simulink model "CounterUpDown_RE_test"  (R2013a)
settings: Solver=ode3  StartTime=0.0  StopTime=10  RelTol=1e-3
libraries: simulink_extras x2, PTC_MBDS_LIB x1
settings Model: Creator=kyle.willis  LastModifiedBy=kyle.willis
settings OptimizationCC: InlineParams=on

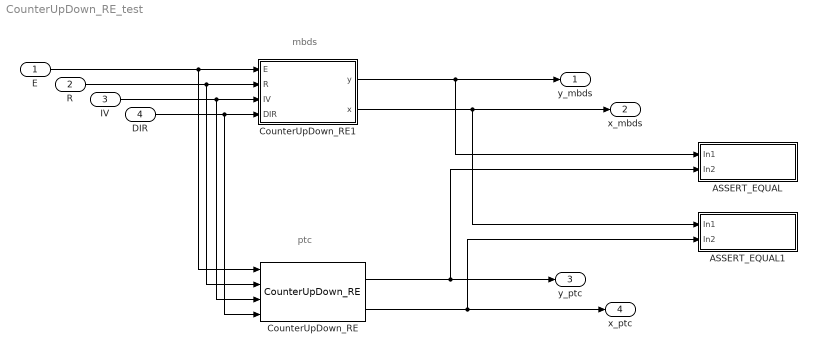
== system CounterUpDown_RE_test ==
  note: ptc
  note: mbds
  E : Inport
  R : Inport  Port=2
  IV : Inport  Port=3
  DIR : Inport  Port=4
  ASSERT_EQUAL : Subsystem
  ASSERT_EQUAL1 : Subsystem
  CounterUpDown_RE : PTC_MBDS_LIB/MBDS Standard Library/Extended Operations/Counter & Timer/CounterUpDown_RE  E_Enabled=on  R_Enabled=on  IV_Enabled=on  IV=0  y_Enabled=on  x_Enabled=on  OutDataTypeStr=Inherit: Inherit via back propagation  PTC_MBDS_BlockVersion=5.40  PTC_BlockType=PTC_MBDS_CounterUpDown_RE
  CounterUpDown_RE1 : Subsystem  InitFcn=|  mask(CounterUpDown_RE){MBDS_LibraryBlock=on, E_Enabled=on, R_Enabled=on, IV_Enabled=on, IV=0, y_Enabled=on, x_Enabled=on, OutDataTypeStr=Inherit: Inherit via back propagation, MBDS_BlockVersion=05.40}
      | if(exist('MBDS_BlockCallback', 'file'))
      |    MBDS_BlockCallback('Update', gcb);
      | end
      mask prompts: MBDS_LibraryBlock "MBDS library block"; E_Enabled "Show E port"; R_Enabled "Show R port"; IV_Enabled "Show IV port"; IV "Initial value (IV):"; y_Enabled "Show y port"; x_Enabled "Show x port"; OutDataTypeStr "Output data type:"; MBDS_BlockVersion "Block version:"
      mask help: This block provides a counter where the direction of counting (up or down) can be controlled by an input port.
      mask init:
      | if(exist('MBDS_BlockCallback', 'file'))
      |    MBDS_BlockCallback('Init', gcb);
      | else
      |    % Disable all mask parameters
      |    MaskEnables = get_param(gcb, 'MaskEnables');
      |    for k = [1:length(MaskEnables)]
      |       MaskEnables{k} = 'off';
      |    end
      |    if(~isequal(MaskEnables, get_param(gcb, 'MaskEnables')))
      |       set_param(gcb, 'MaskEnables', MaskEnables);
      |    end
      | end
      mask Help: eval(['open([workdir(''library_dir:''),''\Blockset\help\'',get_param(gcb,''MaskType''),''.html''])'])
      mask Callback R_Enabled:
      | % Update mask parameter dialog
      | if(exist('MBDS_BlockCallback', 'file'))
      |    MBDS_BlockCallback('R_Enabled', gcb);
      | end
      mask Callback IV_Enabled:
      | % Update mask parameter dialog
      | if(exist('MBDS_BlockCallback', 'file'))
      |    MBDS_BlockCallback('IV_Enabled', gcb);
      | end
      mask Callback IV:
      | % Adopt Value
      | if(exist('MBDS_BlockCallback', 'file'))
      |    MBDS_BlockCallback('IV', gcb);
      | end
      mask Callback y_Enabled:
      | % Update mask parameter dialog
      | if(exist('MBDS_BlockCallback', 'file'))
      |    MBDS_BlockCallback('y_Enabled', gcb);
      | end
      mask Callback x_Enabled:
      | % Update mask parameter dialog
      | if(exist('MBDS_BlockCallback', 'file'))
      |    MBDS_BlockCallback('x_Enabled', gcb);
      | end
      mask TypeOptions OutDataTypeStr: Inherit: Inherit via back propagation | int8 | uint8 | int16 | uint16 | int32 | uint32
      mask Callback OutDataTypeStr:
      | % Configure data type
      | if(exist('MBDS_BlockCallback', 'file'))
      |    MBDS_BlockCallback('OutDataTypeStr', gcb);
      | end
      mask Display:
      | % Show icon or block text
      | if(exist('CounterUpDown.tif', 'file'))
      |    image(imread('CounterUpDown.tif','tif'), [0.295739348370927 0.225 0.378947368421053 0.55]);
      |    disp('')
      | else
      |    disp(sprintf('Count\nUp/Down'));
      | end
      | 
      | % Display port labels
      | port_label('input', 1, 'E');
      | port_label('input', 2, 'R');
      | port_label('input', 3, 'IV');
      | port_label('input', 4, 'DIR');
      | port_label('output', 1, 'y');
      | port_label('output', 2, 'x');
  y_mbds : Outport
  x_mbds : Outport  Port=2
  y_ptc : Outport  Port=3
  x_ptc : Outport  Port=4
  wires:
  E/1 -> CounterUpDown_RE1/1(E), CounterUpDown_RE/1
  R/1 -> CounterUpDown_RE1/2(R), CounterUpDown_RE/2
  IV/1 -> CounterUpDown_RE1/3(IV), CounterUpDown_RE/3
  CounterUpDown_RE1/1(y) -> ASSERT_EQUAL/1(In1), y_mbds/1
  CounterUpDown_RE1/2(x) -> x_mbds/1, ASSERT_EQUAL1/1(In1)
  CounterUpDown_RE/1 -> ASSERT_EQUAL/2(In2), y_ptc/1
  CounterUpDown_RE/2 -> ASSERT_EQUAL1/2(In2), x_ptc/1
  DIR/1 -> CounterUpDown_RE1/4(DIR), CounterUpDown_RE/4

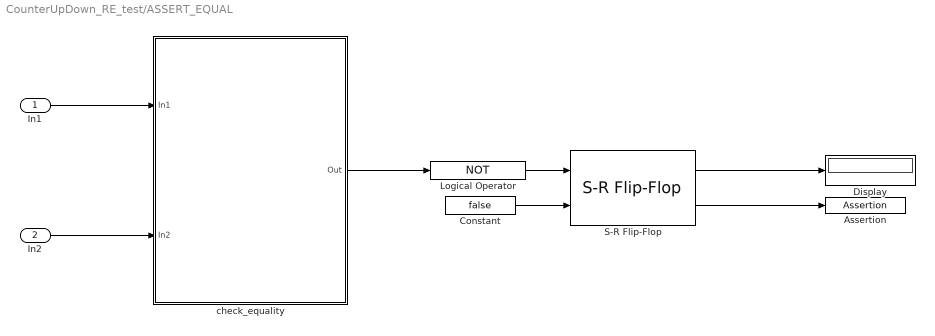
== system CounterUpDown_RE_test/ASSERT_EQUAL ==
  In1 : Inport
  In2 : Inport  Port=2
  Assertion : Assertion
  Constant : Constant  Value=false
  Display : Display
  Logical Operator : Logic  Operator=NOT  AllPortsSameDT=off  OutDataTypeStr=boolean
  S-R Flip-Flop : simulink_extras/Flip Flops/S-R Flip-Flop  initial_condition=0
  check_equality : MATLAB Function  TreatAsAtomicUnit=on
  wires:
  S-R Flip-Flop/1 -> Display/1
  check_equality/1(Out) -> Logical Operator/1
  Constant/1 -> S-R Flip-Flop/2
  S-R Flip-Flop/2 -> Assertion/1
  In2/1 -> check_equality/2(In2)
  In1/1 -> check_equality/1(In1)
  Logical Operator/1 -> S-R Flip-Flop/1

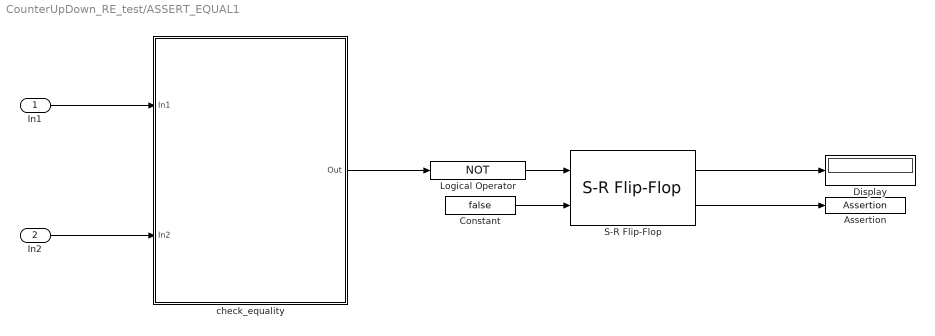
== system CounterUpDown_RE_test/ASSERT_EQUAL1 ==
  In1 : Inport
  In2 : Inport  Port=2
  Assertion : Assertion
  Constant : Constant  Value=false
  Display : Display
  Logical Operator : Logic  Operator=NOT  AllPortsSameDT=off  OutDataTypeStr=boolean
  S-R Flip-Flop : simulink_extras/Flip Flops/S-R Flip-Flop  initial_condition=0
  check_equality : MATLAB Function  TreatAsAtomicUnit=on
  wires:
  Logical Operator/1 -> S-R Flip-Flop/1
  In1/1 -> check_equality/1(In1)
  In2/1 -> check_equality/2(In2)
  S-R Flip-Flop/2 -> Assertion/1
  Constant/1 -> S-R Flip-Flop/2
  check_equality/1(Out) -> Logical Operator/1
  S-R Flip-Flop/1 -> Display/1

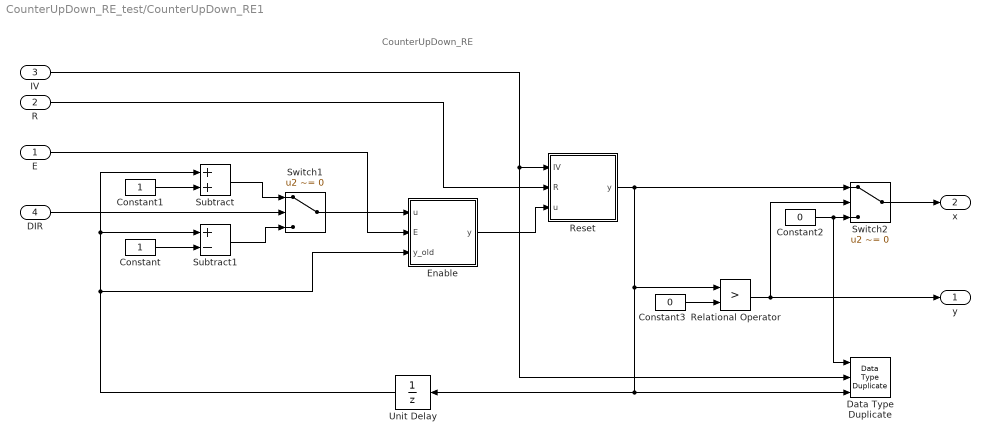
== system CounterUpDown_RE_test/CounterUpDown_RE1 ==
  note: CounterUpDown_RE
  E : Inport  OutDataTypeStr=boolean
  R : Inport  Port=2  OutDataTypeStr=boolean
  IV : Inport  Port=3
  DIR : Inport  Port=4  OutDataTypeStr=boolean
  Constant : Constant  OutDataTypeStr=Inherit: Inherit via back propagation
  Constant1 : Constant  OutDataTypeStr=Inherit: Inherit via back propagation
  Constant2 : Constant  Value=0  OutDataTypeStr=Inherit: Inherit via back propagation
  Constant3 : Constant  Value=0  OutDataTypeStr=Inherit: Inherit via back propagation
  Data Type Duplicate : DataTypeDuplicate  NumInputPorts=3
  Enable : Subsystem
  Relational Operator : RelationalOperator  Operator=>  OutDataTypeStr=boolean  InputSameDT=on
  Reset : Subsystem
  Subtract : Sum  OutDataTypeStr=Inherit: Inherit via back propagation  SaturateOnIntegerOverflow=on  InputSameDT=on
  Subtract1 : Sum  Inputs=+-  OutDataTypeStr=Inherit: Inherit via back propagation  SaturateOnIntegerOverflow=on  InputSameDT=on
  Switch1 : Switch  Criteria=u2 ~= 0  OutDataTypeStr=Inherit: Inherit via back propagation  InputSameDT=on
  Switch2 : Switch  Criteria=u2 ~= 0  OutDataTypeStr=Inherit: Inherit via back propagation  InputSameDT=on
  Unit Delay : UnitDelay  SampleTime=-1
  y : Outport
  x : Outport  Port=2
  wires:
  DIR/1 -> Switch1/2
  R/1 -> Reset/2(R)
  E/1 -> Enable/2(E)
  Subtract/1 -> Switch1/1
  Subtract1/1 -> Switch1/3
  Constant/1 -> Subtract1/2
  Constant1/1 -> Subtract/2
  Switch1/1 -> Enable/1(u)
  Relational Operator/1 -> Switch2/2, y/1
  IV/1 -> Data Type Duplicate/2, Reset/1(IV)
  Switch2/1 -> x/1
  Constant3/1 -> Relational Operator/2
  Constant2/1 -> Switch2/3, Data Type Duplicate/1
  Unit Delay/1 -> Enable/3(y_old), Subtract1/1, Subtract/1
  Reset/1(y) -> Unit Delay/1, Data Type Duplicate/3, Relational Operator/1, Switch2/1
  Enable/1(y) -> Reset/3(u)

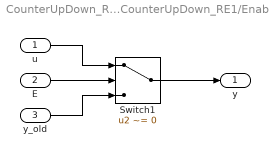
== system CounterUpDown_RE_test/CounterUpDown_RE1/Enable ==
  u : Inport
  E : Inport  Port=2
  y_old : Inport  Port=3
  Switch1 : Switch  Criteria=u2 ~= 0  OutDataTypeStr=Inherit: Inherit via back propagation  InputSameDT=on
  y : Outport
  wires:
  y_old/1 -> Switch1/3
  Switch1/1 -> y/1
  u/1 -> Switch1/1
  E/1 -> Switch1/2

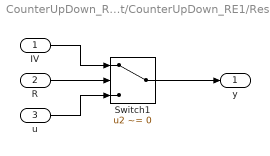
== system CounterUpDown_RE_test/CounterUpDown_RE1/Reset ==
  IV : Inport
  R : Inport  Port=2
  u : Inport  Port=3
  Switch1 : Switch  Criteria=u2 ~= 0  OutDataTypeStr=Inherit: Inherit via back propagation  InputSameDT=on
  y : Outport
  wires:
  u/1 -> Switch1/3
  Switch1/1 -> y/1
  IV/1 -> Switch1/1
  R/1 -> Switch1/2

== matlab function CounterUpDown_RE_test/ASSERT_EQUAL1/check_equality ==
  data: In1 input; Out output; In2 input
function Out = check_equality(In1, In2)
%#codegen

Out = isequaln(In1, In2);

end

== matlab function CounterUpDown_RE_test/ASSERT_EQUAL/check_equality ==
  data: In1 input; Out output; In2 input
function Out = check_equality(In1, In2)
%#codegen

Out = isequaln(In1, In2);

end
